simulink model "ManipRoboticoAdattativoSpazioGiunti"  (R2025b)
settings: Solver=ode45  StartTime=0.0  StopTime=100  MaxStep=1e-3  RelTol=1e-3
values from neighbouring files (symbols this model uses):
  Delta = Kd_mat \ Kp_mat    [main.m]
  Gamma = eye(8) * 20    [main.m]
  Kd = [15; 15]    [main.m]
settings Model: Creator=arman  LastModifiedBy=Armando

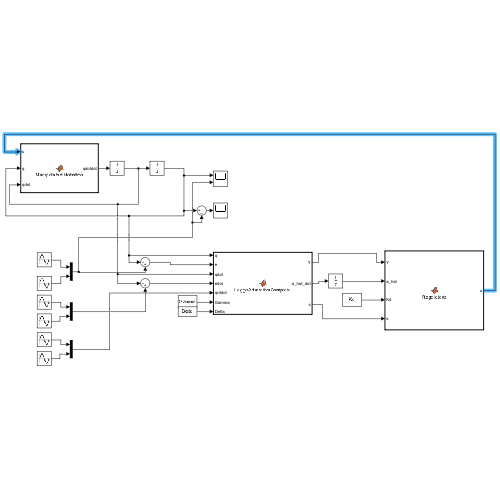
[thumbnail: Simulink's stored preview of the top-level diagram]
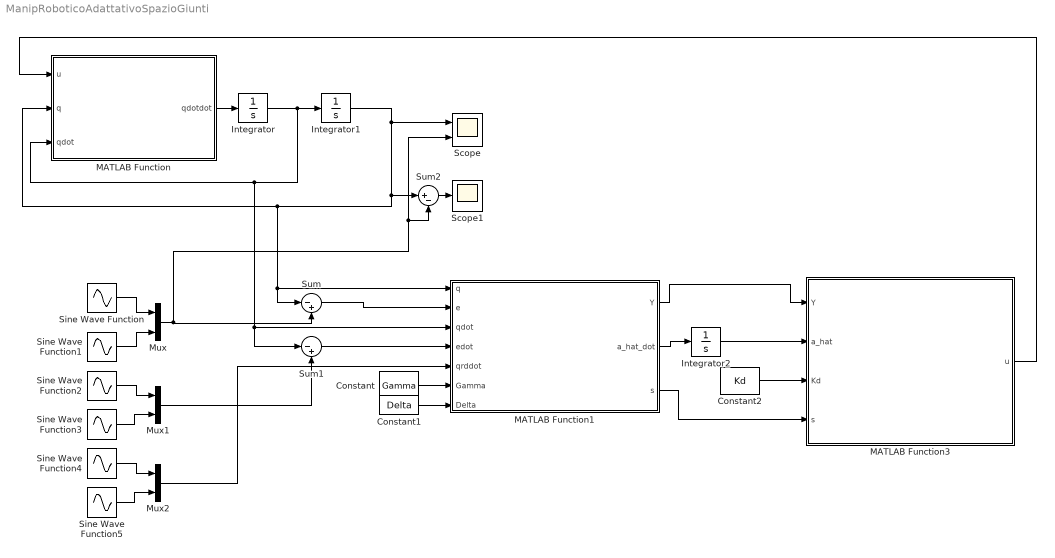
== system ManipRoboticoAdattativoSpazioGiunti ==
  Constant : Constant  Value=Gamma
  Constant1 : Constant  Value=Delta
  Constant2 : Constant  Value=Kd
  Integrator : Integrator  InitialCondition=[0;0]
  Integrator1 : Integrator  InitialCondition=[0;0]
  Integrator2 : Integrator  InitialCondition=[1; 1 ;1 ;1 ;1 ;1 ;1 ;1]
  MATLAB Function : MATLAB Function  TreatAsAtomicUnit=on
  MATLAB Function1 : MATLAB Function  TreatAsAtomicUnit=on
  MATLAB Function3 : MATLAB Function  TreatAsAtomicUnit=on
  Mux : Mux  Inputs=2
  Mux1 : Mux  Inputs=2
  Mux2 : Mux  Inputs=2
  Scope : Scope  NumInputPorts=2
      settings: ActiveDisplayYMinimum=-2.6101607539323664  ActiveDisplayYMaximum=2.5342158467761071
  Scope1 : Scope
      settings: ActiveDisplayYMinimum=-1.6669245640893642  ActiveDisplayYMaximum=0.88680011824504767
  Sine Wave Function : Sin  Amplitude=-1  SampleTime=0
  Sine Wave Function1 : Sin  Amplitude=-2  SampleTime=0
  Sine Wave Function2 : Sin  Amplitude=-1  Phase=pi/2  SampleTime=0
  Sine Wave Function3 : Sin  Amplitude=-2  Phase=pi/2  SampleTime=0
  Sine Wave Function4 : Sin  SampleTime=0
  Sine Wave Function5 : Sin  Amplitude=2  SampleTime=0
  Sum : Sum  Inputs=|-+
  Sum1 : Sum  Inputs=|-+
  Sum2 : Sum  Inputs=|+-
  wires:
  MATLAB Function/1(qdotdot) -> Integrator/1
  Integrator/1 -> MATLAB Function1/3(qdot), Sum1/1, MATLAB Function/3(qdot), Integrator1/1
  Integrator1/1 -> Scope/1, Sum2/1, Sum/1, MATLAB Function1/1(q), MATLAB Function/2(q)
  Sum/1 -> MATLAB Function1/2(e)
  Mux1/1 -> Sum1/2
  Sum1/1 -> MATLAB Function1/4(edot)
  Mux2/1 -> MATLAB Function1/5(qrddot)
  Constant/1 -> MATLAB Function1/6(Gamma)
  Constant1/1 -> MATLAB Function1/7(Delta)
  MATLAB Function1/1(Y) -> MATLAB Function3/1(Y)
  MATLAB Function1/2(a_hat_dot) -> Integrator2/1
  Integrator2/1 -> MATLAB Function3/2(a_hat)
  Constant2/1 -> MATLAB Function3/3(Kd)
  MATLAB Function3/1(u) -> MATLAB Function/1(u)
  Sine Wave Function/1 -> Mux/1
  Sine Wave Function1/1 -> Mux/2
  Mux/1 -> Sum/2, Sum2/2, Scope/2
  Sine Wave Function3/1 -> Mux1/2
  Sine Wave Function2/1 -> Mux1/1
  Sine Wave Function4/1 -> Mux2/1
  Sine Wave Function5/1 -> Mux2/2
  MATLAB Function1/3(s) -> MATLAB Function3/4(s)
  Sum2/1 -> Scope1/1

== matlab function ManipRoboticoAdattativoSpazioGiunti/MATLAB Function1 ==
  data: Y output; q input; e input; qdot input; a_hat_dot output; edot input; qrddot input; Gamma input; Delta input; s output
function [Y, a_hat_dot,s] = LeggeAdattativaCompleta(q, e, qdot, edot, qrddot, Gamma, Delta)

    q1 = q(1);     
    q2 = q(2);
    q1dot = qdot(1); 
    q2dot = qdot(2);
    q1dd_r = qrddot(1); 
    q2dd_r = qrddot(2);

    c2 = cos(q2);
    s2 = sin(q2);

   Y = [
    % u1
    q1dd_r, ...                                           
    q2dd_r, ...                                          
    2*c2*q1dd_r + c2*q2dd_r ...                           
      - 2*q2dot*s2*q1dot - q2dot*s2*q2dot, ...            
    0, ...                                              
    cos(q1), ...                                          
    cos(q1 + q2), ...                                     
    q1dot, ...                                            
    0; ...                                                

    % u2
    0, ...                                                
    q1dd_r, ...                                           
    c2*q1dd_r + q1dot*s2*q1dot, ...                       
    q2dd_r, ...                                           
    0, ...                                               
    cos(q1 + q2), ...                                    
    0, ...                                                
    q2dot ...                                             
];


    s = edot + Delta * e;
    a_hat_dot = Gamma * (Y.' * s);

end

== matlab function ManipRoboticoAdattativoSpazioGiunti/MATLAB Function ==
  data: u input; qdotdot output; q input; qdot input
function qdotdot = ManipolatoreRobotico(u,q,qdot)
[B, C, g, F] = calculateMatrixRobotRR(q,qdot);
qdotdot = B \ (u - (C * qdot) - g - F);

== matlab function ManipRoboticoAdattativoSpazioGiunti/MATLAB Function3 ==
  data: Y input; a_hat input; Kd input; s input; u output
function u = Regolatore(Y, a_hat, Kd, s)

    
    Kd_mat = diag(Kd);  

    % Controllo adattativo PD + modello stimato
    u = Y * a_hat + Kd_mat * s;


end
